simulink model "fsk"  (R2023b)
settings: Solver=VariableStepAuto  StartTime=0.0  StopTime=10.0  RelTol=1e-3
settings Model: Creator=hp  LastModifiedBy=hp

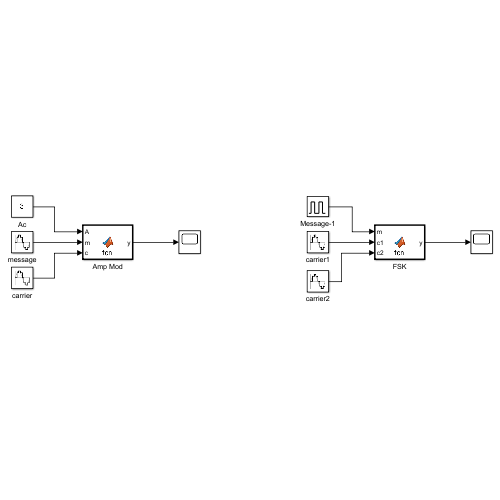
[thumbnail: Simulink's stored preview of the top-level diagram]
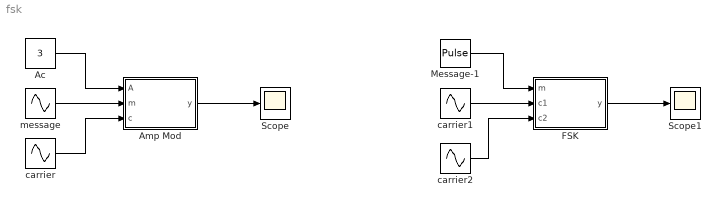
== system fsk ==
  Ac : Constant  Value=3
  Amp Mod : MATLAB Function  TreatAsAtomicUnit=on
  FSK : MATLAB Function  TreatAsAtomicUnit=on
  Message-1 : DiscretePulseGenerator  PulseType=Time based  PulseWidth=50
  Scope : Scope
  Scope1 : Scope
  carrier : Sin  Frequency=20  SampleTime=0.001
  carrier1 : Sin  Frequency=40  SampleTime=0.001
  carrier2 : Sin  Frequency=10  SampleTime=0.001
  message : Sin  Amplitude=3  SampleTime=0.001
  wires:
  Amp Mod/1(y) -> Scope/1
  Ac/1 -> Amp Mod/1(A)
  message/1 -> Amp Mod/2(m)
  carrier/1 -> Amp Mod/3(c)
  Message-1/1 -> FSK/1(m)
  carrier1/1 -> FSK/2(c1)
  FSK/1(y) -> Scope1/1
  carrier2/1 -> FSK/3(c2)

== matlab function fsk/FSK ==
  data: m input; c1 input; y output; c2 input
function y = fcn(m, c1, c2)
 if(m ==1) 
   y = c1;  
 else
   y = c2;
 end

== matlab function fsk/Amp Mod ==
  data: A input; y output; m input; c input
function y = fcn(A, m, c)
y = (A+ m)*c;
